simulink model "mapp_4_fir_4_str"  (R2018b)
settings: Solver=ode45  StartTime=0.0  StopTime=200  RelTol=1e-3  EnableMultiTasking=on
undefined symbols (not defined in the file or in its folder): CMD_ci_Re_0, CMD_ci_Re_21, CMD_ci_str_0, CMD_ci_str_1, CMD_ci_str_10, CMD_ci_str_11, CMD_ci_str_12, CMD_ci_str_13, CMD_ci_str_14, CMD_ci_str_15, CMD_ci_str_16, CMD_ci_str_17, CMD_ci_str_18, CMD_ci_str_19, CMD_ci_str_2, CMD_ci_str_20, CMD_ci_str_21, CMD_ci_str_3, CMD_ci_str_4, CMD_ci_str_5, CMD_ci_str_6, CMD_ci_str_7, CMD_ci_str_8, CMD_ci_str_9, CMD_decr_0, CMD_deka_down, CMD_deka_up, CMD_fb, CMD_FB_mult, CMD_Firprg_0, CMD_Firprg_1, CMD_gain, CMD_ind_mult, CMD_ind_mult_1, CMD_ind_mult_2, CMD_ind_mult_3, CMD_ind_mult_4, CMD_ind_stuk, CMD_ind_vol, CMD_ind_vol_1, CMD_ind_vol_2, CMD_ind_vol_3, CMD_ind_vol_4, CMD_init_dac, CMD_init_sw, CMD_molot_string, CMD_nl, CMD_nl_sl, CMD_omega_0, CMD_out_vol, CMD_param_0, CMD_param_5, CMD_pedal, CMD_reset, CMD_rst, CMD_shape_0, CMD_step_down, CMD_step_up, CMD_str_svertk, ind_mult_0 ... (+10)
libraries: xbsIndex_r4 x3300
(part 15 of 16)

== system mapp_4_fir_4_str/Mid_Graph2/Exp/exp-mashinka/gauss2/exp_e0 ==
  addr : Inport
  m_data : Inport  Port=2
  m_addr : Inport  Port=3
  m_en : Inport  Port=4
  Force_vol : Inport  Port=5
  AddSub5 : xbsIndex_r4/AddSub  mode=Subtraction  use_carryin=off  use_carryout=off  en=off  latency=2  precision=Full  arith_type="Signed  (2's comp)"  n_bits=24  bin_pt=0  quantization=Truncate  overflow=Wrap  use_behavioral_HDL=off  hw_selection=Fabric  pipelined=off  dbl_ovrd=off  block_type=addsub
  AddSub6 : xbsIndex_r4/AddSub  mode=Addition  use_carryin=off  use_carryout=off  en=off  latency=2  precision=Full  arith_type=Unsigned  n_bits=24  bin_pt=0  quantization=Truncate  overflow=Wrap  use_behavioral_HDL=off  hw_selection=Fabric  pipelined=off  dbl_ovrd=off  block_type=addsub
  Constant : xbsIndex_r4/Constant  const=4  gui_display_data_type=Fixed-point  arith_type=Unsigned  n_bits=3  bin_pt=0  preci_type=Single  exp_width=8  frac_width=24  explicit_period=off  period=1  equ=P=C  opselect=C  inp2=PCIN>>17  opr=+  inp1=P  carry=CIN  dbl_ovrd=off  block_type=constant
  Constant1 : xbsIndex_r4/Constant  const=0  gui_display_data_type=Fixed-point  arith_type=Unsigned  n_bits=24  bin_pt=0  preci_type=Single  exp_width=8  frac_width=24  explicit_period=on  period=1  equ=P=C  opselect=C  inp2=PCIN>>17  opr=+  inp1=P  carry=CIN  dbl_ovrd=off  block_type=constant
      settings: block_version=VER_STRING_GOES_HERE
  Constant10 : xbsIndex_r4/Constant  const=0  gui_display_data_type=Fixed-point  arith_type=Unsigned  n_bits=24  bin_pt=0  preci_type=Single  exp_width=8  frac_width=24  explicit_period=on  period=1  equ=P=C  opselect=C  inp2=PCIN>>17  opr=+  inp1=P  carry=CIN  dbl_ovrd=off  block_type=constant
      settings: block_version=VER_STRING_GOES_HERE
  Constant2 : xbsIndex_r4/Constant  const=4  gui_display_data_type=Fixed-point  arith_type=Unsigned  n_bits=3  bin_pt=0  preci_type=Single  exp_width=8  frac_width=24  explicit_period=on  period=1  equ=P=C  opselect=C  inp2=PCIN>>17  opr=+  inp1=P  carry=CIN  dbl_ovrd=off  block_type=constant
      settings: block_version=VER_STRING_GOES_HERE
  Constant3 : xbsIndex_r4/Constant  const=3  gui_display_data_type=Fixed-point  arith_type=Unsigned  n_bits=3  bin_pt=0  preci_type=Single  exp_width=8  frac_width=24  explicit_period=off  period=1  equ=P=C  opselect=C  inp2=PCIN>>17  opr=+  inp1=P  carry=CIN  dbl_ovrd=off  block_type=constant
  Constant4 : xbsIndex_r4/Constant  const=2  gui_display_data_type=Fixed-point  arith_type=Unsigned  n_bits=3  bin_pt=0  preci_type=Single  exp_width=8  frac_width=24  explicit_period=off  period=1  equ=P=C  opselect=C  inp2=PCIN>>17  opr=+  inp1=P  carry=CIN  dbl_ovrd=off  block_type=constant
  Constant5 : xbsIndex_r4/Constant  const=1  gui_display_data_type=Fixed-point  arith_type=Unsigned  n_bits=3  bin_pt=0  preci_type=Single  exp_width=8  frac_width=24  explicit_period=off  period=1  equ=P=C  opselect=C  inp2=PCIN>>17  opr=+  inp1=P  carry=CIN  dbl_ovrd=off  block_type=constant
  Constant6 : xbsIndex_r4/Constant  const=0  gui_display_data_type=Fixed-point  arith_type=Unsigned  n_bits=3  bin_pt=0  preci_type=Single  exp_width=8  frac_width=24  explicit_period=off  period=1  equ=P=C  opselect=C  inp2=PCIN>>17  opr=+  inp1=P  carry=CIN  dbl_ovrd=off  block_type=constant
  Convert5 : xbsIndex_r4/Convert  gui_display_data_type=Fixed-point  arith_type=Unsigned  n_bits=3  bin_pt=0  float_type=Single  exp_bits=8  fraction_bits=24  quantization=Truncate  overflow=Wrap  en=off  latency=0  pipeline=off  dbl_ovrd=off  block_type=convert
  Logical{,1..4} (5 alike) : xbsIndex_r4/Logical  logical_function=AND  inputs=2  en=off  latency=1  precision=Full  arith_type=Unsigned  n_bits=16  bin_pt=0  align_bp=on  dbl_ovrd=off  block_type=logical
  Mult3 : xbsIndex_r4/Mult  precision=Full  arith_type="Signed  (2's comp)"  n_bits=16  bin_pt=14  quantization=Truncate  overflow=Wrap  en=off  latency=3  use_behavioral_HDL=off  opt=Speed  use_embedded=on  optimum_pipeline=off  pipeline=on  dbl_ovrd=off  use_rpm=on  placement_style=Triangular  block_type=mult
  Mux{10..14} (5 alike) : xbsIndex_r4/Mux  inputs=2  en=off  latency=0  precision=Full  arith_type=Unsigned  n_bits=16  bin_pt=14  quantization=Truncate  overflow=Wrap  dbl_ovrd=off  block_type=mux
  Mux2 : xbsIndex_r4/Mux  inputs=2  en=off  latency=1  precision=Full  arith_type=Unsigned  n_bits=16  bin_pt=14  quantization=Truncate  overflow=Wrap  dbl_ovrd=off  block_type=mux
  Mux3 : xbsIndex_r4/Mux  inputs=5  en=off  latency=1  precision=Full  arith_type=Unsigned  n_bits=16  bin_pt=14  quantization=Truncate  overflow=Wrap  dbl_ovrd=off  block_type=mux
  Mux4 : xbsIndex_r4/Mux  inputs=5  en=off  latency=1  precision=Full  arith_type=Unsigned  n_bits=16  bin_pt=14  quantization=Truncate  overflow=Wrap  dbl_ovrd=off  block_type=mux
  RSlice1 : xbsIndex_r4/Slice  nbits=3  boolean_output=off  mode=Upper Bit Location + Width  bit1=0  base1=MSB of Input  bit0=0  base0=LSB of Input  dbl_ovrd=off  block_type=slice
      settings: block_version=VER_STRING_GOES_HERE
  RSlice7 : xbsIndex_r4/Slice  nbits=7  boolean_output=off  mode=Lower Bit Location + Width  bit1=0  base1=MSB of Input  bit0=0  base0=LSB of Input  dbl_ovrd=off  block_type=slice
      settings: block_version=VER_STRING_GOES_HERE
  Relational{1..5,16..17} (7 alike) : xbsIndex_r4/Relational  mode=a=b  op_type=Bool  en=off  latency=0  dbl_ovrd=off  block_type=relational
  Scope1 : Scope  NumInputPorts=8
  Scope2 : Scope  NumInputPorts=8
  Scope3 : Scope  NumInputPorts=10
  Shift2 : xbsIndex_r4/Shift  shift_dir=Right  shift_bits=5  en=off  latency=0  precision=Full  arith_type="Signed  (2's comp)"  n_bits=16  bin_pt=14  quantization=Truncate  overflow=Wrap  dbl_ovrd=off  block_type=shift
  Single Port RAM5 : xbsIndex_r4/Single Port RAM  depth=96  initVector=exp_e4  distributed_mem=Block RAM  write_mode=Read After Write  rst=off  init_reg=0  en=off  latency=1  optimize=Area  dbl_ovrd=off  block_type=spram
  Single Port RAM6 : xbsIndex_r4/Single Port RAM  depth=96  initVector=exp_e3  distributed_mem=Block RAM  write_mode=Read After Write  rst=off  init_reg=0  en=off  latency=1  optimize=Area  dbl_ovrd=off  block_type=spram
  Single Port RAM7 : xbsIndex_r4/Single Port RAM  depth=96  initVector=exp_e2  distributed_mem=Block RAM  write_mode=Read After Write  rst=off  init_reg=0  en=off  latency=1  optimize=Area  dbl_ovrd=off  block_type=spram
  Single Port RAM8 : xbsIndex_r4/Single Port RAM  depth=96  initVector=exp_e1  distributed_mem=Block RAM  write_mode=Read After Write  rst=off  init_reg=0  en=off  latency=1  optimize=Area  dbl_ovrd=off  block_type=spram
  Single Port RAM9 : xbsIndex_r4/Single Port RAM  depth=96  initVector=exp_e0  distributed_mem=Block RAM  write_mode=Read After Write  rst=off  init_reg=0  en=off  latency=1  optimize=Area  dbl_ovrd=off  block_type=spram
  Slice1 : xbsIndex_r4/Slice  nbits=5  boolean_output=off  mode=Lower Bit Location + Width  bit1=0  base1=LSB of Input  bit0=0  base0=LSB of Input  dbl_ovrd=off  block_type=slice
  Slice3 : xbsIndex_r4/Slice  nbits=2  boolean_output=off  mode=Upper Bit Location + Width  bit1=0  base1=MSB of Input  bit0=0  base0=LSB of Input  dbl_ovrd=off  block_type=slice
  const : xbsIndex_r4/Constant  const=0  gui_display_data_type=Fixed-point  arith_type=Unsigned  n_bits=7  bin_pt=0  preci_type=Single  exp_width=8  frac_width=24  explicit_period=on  period=1  equ=P=C  opselect=C  inp2=PCIN>>17  opr=+  inp1=P  carry=CIN  dbl_ovrd=off  block_type=constant
      settings: block_version=VER_STRING_GOES_HERE
  ind_vol_3 : xbsIndex_r4/Constant  const=CMD_ind_vol_3  gui_display_data_type=Fixed-point  arith_type=Unsigned  n_bits=8  bin_pt=0  preci_type=Single  exp_width=8  frac_width=24  explicit_period=on  period=1  equ=P=C  opselect=C  inp2=PCIN>>17  opr=+  inp1=P  carry=CIN  dbl_ovrd=off  block_type=constant
      settings: block_version=VER_STRING_GOES_HERE
  x : xbsIndex_r4/Constant  const=8000000  gui_display_data_type=Fixed-point  arith_type=Unsigned  n_bits=24  bin_pt=0  preci_type=Single  exp_width=8  frac_width=24  explicit_period=on  period=1  equ=P=C  opselect=C  inp2=PCIN>>17  opr=+  inp1=P  carry=CIN  dbl_ovrd=off  block_type=constant
      settings: block_version=VER_STRING_GOES_HERE
  z1 : xbsIndex_r4/Delay  rst=off  infoeditControl=Selection of Reset will increase slice count due to use of real FFs and instead of SRLs  en=off  latency=3  reg_retiming=on  dbl_ovrd=off  block_type=delay
      settings: block_version=8.2-EVAL
  z{2,4..13,15,17..18,20..24} (19 alike) : xbsIndex_r4/Delay  rst=off  infoeditControl=Selection of Reset will increase slice count due to use of real FFs and instead of SRLs  en=off  latency=1  reg_retiming=on  dbl_ovrd=off  block_type=delay
      settings: block_version=8.2-EVAL
  z14 : xbsIndex_r4/Delay  rst=off  infoeditControl=Selection of Reset will increase slice count due to use of real FFs and instead of SRLs  en=off  latency=2  reg_retiming=on  dbl_ovrd=off  block_type=delay
      settings: block_version=8.2-EVAL
  z3 : xbsIndex_r4/Delay  rst=off  infoeditControl=Selection of Reset will increase slice count due to use of real FFs and instead of SRLs  en=off  latency=4  reg_retiming=on  dbl_ovrd=off  block_type=delay
      settings: block_version=8.2-EVAL
  Out : Outport
  wires:
  z17/1 -> Scope1/8, Out/1
  z24/1 -> Scope1/7, AddSub6/2
  z23/1 -> Shift2/1
  z22/1 -> z21/1
  Slice1/1 -> z22/1
  z21/1 -> z20/1
  Mux2/1 -> z18/1
  z18/1 -> Scope3/1, Mux3/1, Mux4/1
  z3/1 -> z24/1
  Mux14/1 -> Single Port RAM9/1
  z4/1 -> z5/1, z6/1, z8/1, z9/1, z7/1
  Relational1/1 -> Logical/2
  Relational2/1 -> Logical1/2
  Constant1/1 -> Mux4/6
  Convert5/1 -> Mux2/2
  Mult3/1 -> z2/1
  z13/1 -> Scope3/2, Mux3/2, Mux4/3
  Relational16/1 -> Mux2/1
  Single Port RAM7/1 -> z12/1
  Single Port RAM6/1 -> z11/1
  z15/1 -> Mux4/2
  Relational5/1 -> Logical4/2
  Constant6/1 -> Relational5/2
  RSlice7/1 -> Mux10/3, Mux13/3, Mux14/3, Mux12/3, Mux11/3
  Relational17/1 -> Logical1/1, Logical2/1, Logical3/1, Logical4/1, Logical/1
  Logical1/1 -> Mux11/1, Single Port RAM6/3
  Relational3/1 -> Logical2/2
  Constant5/1 -> Relational4/2
  Slice3/1 -> Convert5/1
  Mux3/1 -> AddSub5/1, Scope3/6
  Mux12/1 -> Single Port RAM7/1
  z7/1 -> Mux12/2
  Constant4/1 -> Relational3/2
  Shift2/1 -> Scope1/3, Mult3/1
  z14/1 -> z3/1
  Mux13/1 -> Single Port RAM8/1
  m_data/1 -> Single Port RAM8/2, Single Port RAM9/2, Single Port RAM7/2, Single Port RAM6/2, Single Port RAM5/2
  Mux10/1 -> Single Port RAM5/1, Scope2/1
  z5/1 -> Mux10/2
  z6/1 -> Mux11/2
  ind_vol_3/1 -> Relational17/2
  z8/1 -> Mux13/2
  Single Port RAM5/1 -> z10/1, Scope2/3
  Constant3/1 -> Relational2/2
  Mux11/1 -> Single Port RAM6/1
  z9/1 -> Mux14/2
  Relational4/1 -> Logical3/2
  RSlice1/1 -> Relational2/1, Relational3/1, Relational4/1, Relational5/1, Relational1/1
  Logical4/1 -> Mux14/1, Single Port RAM9/3
  addr/1 -> z4/1
  Mux4/1 -> AddSub5/2, Scope3/7, z14/1
  AddSub5/1 -> z23/1
  const/1 -> Relational16/2
  z1/1 -> Scope1/4, Mult3/2
  Logical/1 -> Mux10/1, Single Port RAM5/3, Scope2/2
  Constant10/1 -> Mux3/6
  Constant/1 -> Relational1/2
  Single Port RAM9/1 -> z15/1
  z20/1 -> Scope1/2, z1/1
  Force_vol/1 -> Slice3/1, Scope1/1, Slice1/1, Relational16/1
  Logical3/1 -> Single Port RAM8/3, Mux13/1
  Single Port RAM8/1 -> z13/1
  z2/1 -> Scope1/6, AddSub6/1
  Logical2/1 -> Mux12/1, Single Port RAM7/3
  Constant2/1 -> Mux2/3
  z10/1 -> Scope3/5, Mux3/5
  m_addr/1 -> RSlice1/1, RSlice7/1
  z11/1 -> Scope3/4, Mux3/4, Mux4/5
  z12/1 -> Mux4/4, Scope3/3, Mux3/3
  m_en/1 -> Relational17/1
  AddSub6/1 -> z17/1

== system mapp_4_fir_4_str/Mid_Graph2/Exp/exp-mashinka/gauss3/exp_a0 ==
  addr : Inport
  m_data : Inport  Port=2
  m_addr : Inport  Port=3
  m_en : Inport  Port=4
  Force_vol : Inport  Port=5
  AddSub5 : xbsIndex_r4/AddSub  mode=Subtraction  use_carryin=off  use_carryout=off  en=off  latency=2  precision=Full  arith_type="Signed  (2's comp)"  n_bits=24  bin_pt=0  quantization=Truncate  overflow=Wrap  use_behavioral_HDL=off  hw_selection=Fabric  pipelined=off  dbl_ovrd=off  block_type=addsub
  AddSub6 : xbsIndex_r4/AddSub  mode=Addition  use_carryin=off  use_carryout=off  en=off  latency=2  precision=Full  arith_type=Unsigned  n_bits=24  bin_pt=0  quantization=Truncate  overflow=Wrap  use_behavioral_HDL=off  hw_selection=Fabric  pipelined=off  dbl_ovrd=off  block_type=addsub
  CMD_step_down : xbsIndex_r4/Constant  const=CMD_step_down  gui_display_data_type=Fixed-point  arith_type=Unsigned  n_bits=8  bin_pt=0  preci_type=Single  exp_width=8  frac_width=24  explicit_period=on  period=1  equ=P=C  opselect=C  inp2=PCIN>>17  opr=+  inp1=P  carry=CIN  dbl_ovrd=off  block_type=constant
      settings: block_version=VER_STRING_GOES_HERE
  Constant : xbsIndex_r4/Constant  const=4  gui_display_data_type=Fixed-point  arith_type=Unsigned  n_bits=3  bin_pt=0  preci_type=Single  exp_width=8  frac_width=24  explicit_period=off  period=1  equ=P=C  opselect=C  inp2=PCIN>>17  opr=+  inp1=P  carry=CIN  dbl_ovrd=off  block_type=constant
  Constant1 : xbsIndex_r4/Constant  const=0  gui_display_data_type=Fixed-point  arith_type=Unsigned  n_bits=24  bin_pt=0  preci_type=Single  exp_width=8  frac_width=24  explicit_period=on  period=1  equ=P=C  opselect=C  inp2=PCIN>>17  opr=+  inp1=P  carry=CIN  dbl_ovrd=off  block_type=constant
      settings: block_version=VER_STRING_GOES_HERE
  Constant10 : xbsIndex_r4/Constant  const=0  gui_display_data_type=Fixed-point  arith_type=Unsigned  n_bits=24  bin_pt=0  preci_type=Single  exp_width=8  frac_width=24  explicit_period=on  period=1  equ=P=C  opselect=C  inp2=PCIN>>17  opr=+  inp1=P  carry=CIN  dbl_ovrd=off  block_type=constant
      settings: block_version=VER_STRING_GOES_HERE
  Constant2 : xbsIndex_r4/Constant  const=4  gui_display_data_type=Fixed-point  arith_type=Unsigned  n_bits=3  bin_pt=0  preci_type=Single  exp_width=8  frac_width=24  explicit_period=on  period=1  equ=P=C  opselect=C  inp2=PCIN>>17  opr=+  inp1=P  carry=CIN  dbl_ovrd=off  block_type=constant
      settings: block_version=VER_STRING_GOES_HERE
  Constant3 : xbsIndex_r4/Constant  const=3  gui_display_data_type=Fixed-point  arith_type=Unsigned  n_bits=3  bin_pt=0  preci_type=Single  exp_width=8  frac_width=24  explicit_period=off  period=1  equ=P=C  opselect=C  inp2=PCIN>>17  opr=+  inp1=P  carry=CIN  dbl_ovrd=off  block_type=constant
  Constant4 : xbsIndex_r4/Constant  const=2  gui_display_data_type=Fixed-point  arith_type=Unsigned  n_bits=3  bin_pt=0  preci_type=Single  exp_width=8  frac_width=24  explicit_period=off  period=1  equ=P=C  opselect=C  inp2=PCIN>>17  opr=+  inp1=P  carry=CIN  dbl_ovrd=off  block_type=constant
  Constant5 : xbsIndex_r4/Constant  const=1  gui_display_data_type=Fixed-point  arith_type=Unsigned  n_bits=3  bin_pt=0  preci_type=Single  exp_width=8  frac_width=24  explicit_period=off  period=1  equ=P=C  opselect=C  inp2=PCIN>>17  opr=+  inp1=P  carry=CIN  dbl_ovrd=off  block_type=constant
  Constant6 : xbsIndex_r4/Constant  const=0  gui_display_data_type=Fixed-point  arith_type=Unsigned  n_bits=3  bin_pt=0  preci_type=Single  exp_width=8  frac_width=24  explicit_period=off  period=1  equ=P=C  opselect=C  inp2=PCIN>>17  opr=+  inp1=P  carry=CIN  dbl_ovrd=off  block_type=constant
  Convert5 : xbsIndex_r4/Convert  gui_display_data_type=Fixed-point  arith_type=Unsigned  n_bits=3  bin_pt=0  float_type=Single  exp_bits=8  fraction_bits=24  quantization=Truncate  overflow=Wrap  en=off  latency=0  pipeline=off  dbl_ovrd=off  block_type=convert
  Logical{,1..4} (5 alike) : xbsIndex_r4/Logical  logical_function=AND  inputs=2  en=off  latency=1  precision=Full  arith_type=Unsigned  n_bits=16  bin_pt=0  align_bp=on  dbl_ovrd=off  block_type=logical
  Mult3 : xbsIndex_r4/Mult  precision=Full  arith_type="Signed  (2's comp)"  n_bits=16  bin_pt=14  quantization=Truncate  overflow=Wrap  en=off  latency=3  use_behavioral_HDL=off  opt=Speed  use_embedded=on  optimum_pipeline=off  pipeline=on  dbl_ovrd=off  use_rpm=on  placement_style=Triangular  block_type=mult
  Mux{10..14} (5 alike) : xbsIndex_r4/Mux  inputs=2  en=off  latency=0  precision=Full  arith_type=Unsigned  n_bits=16  bin_pt=14  quantization=Truncate  overflow=Wrap  dbl_ovrd=off  block_type=mux
  Mux2 : xbsIndex_r4/Mux  inputs=2  en=off  latency=1  precision=Full  arith_type=Unsigned  n_bits=16  bin_pt=14  quantization=Truncate  overflow=Wrap  dbl_ovrd=off  block_type=mux
  Mux3 : xbsIndex_r4/Mux  inputs=5  en=off  latency=1  precision=Full  arith_type=Unsigned  n_bits=16  bin_pt=14  quantization=Truncate  overflow=Wrap  dbl_ovrd=off  block_type=mux
  Mux4 : xbsIndex_r4/Mux  inputs=5  en=off  latency=1  precision=Full  arith_type=Unsigned  n_bits=16  bin_pt=14  quantization=Truncate  overflow=Wrap  dbl_ovrd=off  block_type=mux
  RSlice1 : xbsIndex_r4/Slice  nbits=3  boolean_output=off  mode=Upper Bit Location + Width  bit1=0  base1=MSB of Input  bit0=0  base0=LSB of Input  dbl_ovrd=off  block_type=slice
      settings: block_version=VER_STRING_GOES_HERE
  RSlice7 : xbsIndex_r4/Slice  nbits=7  boolean_output=off  mode=Lower Bit Location + Width  bit1=0  base1=MSB of Input  bit0=0  base0=LSB of Input  dbl_ovrd=off  block_type=slice
      settings: block_version=VER_STRING_GOES_HERE
  Relational{1..5,16..17} (7 alike) : xbsIndex_r4/Relational  mode=a=b  op_type=Bool  en=off  latency=0  dbl_ovrd=off  block_type=relational
  Scope1 : Scope  NumInputPorts=8
  Scope2 : Scope  NumInputPorts=8
  Scope3 : Scope  NumInputPorts=10
  Shift2 : xbsIndex_r4/Shift  shift_dir=Right  shift_bits=5  en=off  latency=0  precision=Full  arith_type="Signed  (2's comp)"  n_bits=16  bin_pt=14  quantization=Truncate  overflow=Wrap  dbl_ovrd=off  block_type=shift
  Single Port RAM5 : xbsIndex_r4/Single Port RAM  depth=96  initVector=exp_a4  distributed_mem=Block RAM  write_mode=Read After Write  rst=off  init_reg=0  en=off  latency=1  optimize=Area  dbl_ovrd=off  block_type=spram
  Single Port RAM6 : xbsIndex_r4/Single Port RAM  depth=96  initVector=exp_a3  distributed_mem=Block RAM  write_mode=Read After Write  rst=off  init_reg=0  en=off  latency=1  optimize=Area  dbl_ovrd=off  block_type=spram
  Single Port RAM7 : xbsIndex_r4/Single Port RAM  depth=96  initVector=exp_a2  distributed_mem=Block RAM  write_mode=Read After Write  rst=off  init_reg=0  en=off  latency=1  optimize=Area  dbl_ovrd=off  block_type=spram
  Single Port RAM8 : xbsIndex_r4/Single Port RAM  depth=96  initVector=exp_a1  distributed_mem=Block RAM  write_mode=Read After Write  rst=off  init_reg=0  en=off  latency=1  optimize=Area  dbl_ovrd=off  block_type=spram
  Single Port RAM9 : xbsIndex_r4/Single Port RAM  depth=96  initVector=exp_a0  distributed_mem=Block RAM  write_mode=Read After Write  rst=off  init_reg=0  en=off  latency=1  optimize=Area  dbl_ovrd=off  block_type=spram
  Slice1 : xbsIndex_r4/Slice  nbits=5  boolean_output=off  mode=Lower Bit Location + Width  bit1=0  base1=LSB of Input  bit0=0  base0=LSB of Input  dbl_ovrd=off  block_type=slice
  Slice3 : xbsIndex_r4/Slice  nbits=2  boolean_output=off  mode=Upper Bit Location + Width  bit1=0  base1=MSB of Input  bit0=0  base0=LSB of Input  dbl_ovrd=off  block_type=slice
  const : xbsIndex_r4/Constant  const=0  gui_display_data_type=Fixed-point  arith_type=Unsigned  n_bits=7  bin_pt=0  preci_type=Single  exp_width=8  frac_width=24  explicit_period=on  period=1  equ=P=C  opselect=C  inp2=PCIN>>17  opr=+  inp1=P  carry=CIN  dbl_ovrd=off  block_type=constant
      settings: block_version=VER_STRING_GOES_HERE
  x : xbsIndex_r4/Constant  const=8000000  gui_display_data_type=Fixed-point  arith_type=Unsigned  n_bits=24  bin_pt=0  preci_type=Single  exp_width=8  frac_width=24  explicit_period=on  period=1  equ=P=C  opselect=C  inp2=PCIN>>17  opr=+  inp1=P  carry=CIN  dbl_ovrd=off  block_type=constant
      settings: block_version=VER_STRING_GOES_HERE
  z1 : xbsIndex_r4/Delay  rst=off  infoeditControl=Selection of Reset will increase slice count due to use of real FFs and instead of SRLs  en=off  latency=3  reg_retiming=on  dbl_ovrd=off  block_type=delay
      settings: block_version=8.2-EVAL
  z{2,4..13,15,17..18,20..24} (19 alike) : xbsIndex_r4/Delay  rst=off  infoeditControl=Selection of Reset will increase slice count due to use of real FFs and instead of SRLs  en=off  latency=1  reg_retiming=on  dbl_ovrd=off  block_type=delay
      settings: block_version=8.2-EVAL
  z14 : xbsIndex_r4/Delay  rst=off  infoeditControl=Selection of Reset will increase slice count due to use of real FFs and instead of SRLs  en=off  latency=2  reg_retiming=on  dbl_ovrd=off  block_type=delay
      settings: block_version=8.2-EVAL
  z3 : xbsIndex_r4/Delay  rst=off  infoeditControl=Selection of Reset will increase slice count due to use of real FFs and instead of SRLs  en=off  latency=4  reg_retiming=on  dbl_ovrd=off  block_type=delay
      settings: block_version=8.2-EVAL
  Out : Outport
  wires:
  AddSub6/1 -> z17/1
  m_en/1 -> Relational17/1
  z12/1 -> Mux3/3, Scope3/3, Mux4/4
  z11/1 -> Mux4/5, Mux3/4, Scope3/4
  m_addr/1 -> RSlice7/1, RSlice1/1
  z10/1 -> Mux3/5, Scope3/5
  Constant2/1 -> Mux2/3
  Logical2/1 -> Single Port RAM7/3, Mux12/1
  z2/1 -> Scope1/4, AddSub6/1
  Single Port RAM8/1 -> z13/1
  Logical3/1 -> Mux13/1, Single Port RAM8/3
  Force_vol/1 -> Relational16/1, Slice1/1, Slice3/1
  z20/1 -> z1/1
  Single Port RAM9/1 -> z15/1
  Constant/1 -> Relational1/2
  Constant10/1 -> Mux3/6
  Logical/1 -> Scope2/2, Single Port RAM5/3, Mux10/1
  z1/1 -> Scope1/3, Mult3/2
  const/1 -> Relational16/2
  AddSub5/1 -> z23/1
  Mux4/1 -> z14/1, Scope3/7, AddSub5/2
  addr/1 -> z4/1
  Logical4/1 -> Single Port RAM9/3, Mux14/1
  RSlice1/1 -> Relational1/1, Relational5/1, Relational4/1, Relational3/1, Relational2/1
  Relational4/1 -> Logical3/2
  z9/1 -> Mux14/2
  Mux11/1 -> Single Port RAM6/1
  Constant3/1 -> Relational2/2
  Single Port RAM5/1 -> Scope2/3, z10/1
  z8/1 -> Mux13/2
  CMD_step_down/1 -> Relational17/2
  z6/1 -> Mux11/2
  z5/1 -> Mux10/2
  Mux10/1 -> Scope2/1, Single Port RAM5/1
  m_data/1 -> Single Port RAM5/2, Single Port RAM6/2, Single Port RAM7/2, Single Port RAM9/2, Single Port RAM8/2
  Mux13/1 -> Single Port RAM8/1
  z14/1 -> z3/1
  Shift2/1 -> Scope1/1, Mult3/1
  Constant4/1 -> Relational3/2
  z7/1 -> Mux12/2
  Mux12/1 -> Single Port RAM7/1
  Mux3/1 -> Scope3/6, AddSub5/1
  Slice3/1 -> Convert5/1
  Constant5/1 -> Relational4/2
  Relational3/1 -> Logical2/2
  Logical1/1 -> Single Port RAM6/3, Mux11/1
  Relational17/1 -> Logical/1, Logical4/1, Logical3/1, Logical2/1, Logical1/1
  RSlice7/1 -> Mux11/3, Mux12/3, Mux14/3, Mux13/3, Mux10/3
  Constant6/1 -> Relational5/2
  Relational5/1 -> Logical4/2
  z15/1 -> Mux4/2
  Single Port RAM6/1 -> z11/1
  Single Port RAM7/1 -> z12/1
  Relational16/1 -> Mux2/1
  z13/1 -> Mux4/3, Mux3/2, Scope3/2
  Mult3/1 -> z2/1
  Convert5/1 -> Mux2/2
  Constant1/1 -> Mux4/6
  Relational2/1 -> Logical1/2
  Relational1/1 -> Logical/2
  z4/1 -> z7/1, z9/1, z8/1, z6/1, z5/1
  Mux14/1 -> Single Port RAM9/1
  z3/1 -> z24/1
  z18/1 -> Mux4/1, Mux3/1, Scope3/1
  Mux2/1 -> z18/1
  z21/1 -> z20/1
  Slice1/1 -> z22/1
  z22/1 -> z21/1
  z23/1 -> Shift2/1
  z24/1 -> Scope1/5, AddSub6/2
  z17/1 -> Scope1/6, Out/1

== system mapp_4_fir_4_str/Mid_Graph2/Exp/exp-mashinka/gauss3/exp_d0 ==
  addr : Inport
  m_data : Inport  Port=2
  m_addr : Inport  Port=3
  m_en : Inport  Port=4
  Force_vol : Inport  Port=5
  AddSub5 : xbsIndex_r4/AddSub  mode=Subtraction  use_carryin=off  use_carryout=off  en=off  latency=2  precision=Full  arith_type="Signed  (2's comp)"  n_bits=24  bin_pt=0  quantization=Truncate  overflow=Wrap  use_behavioral_HDL=off  hw_selection=Fabric  pipelined=off  dbl_ovrd=off  block_type=addsub
  AddSub6 : xbsIndex_r4/AddSub  mode=Addition  use_carryin=off  use_carryout=off  en=off  latency=2  precision=Full  arith_type=Unsigned  n_bits=24  bin_pt=0  quantization=Truncate  overflow=Wrap  use_behavioral_HDL=off  hw_selection=Fabric  pipelined=off  dbl_ovrd=off  block_type=addsub
  CMD_step_up : xbsIndex_r4/Constant  const=CMD_step_up  gui_display_data_type=Fixed-point  arith_type=Unsigned  n_bits=8  bin_pt=0  preci_type=Single  exp_width=8  frac_width=24  explicit_period=on  period=1  equ=P=C  opselect=C  inp2=PCIN>>17  opr=+  inp1=P  carry=CIN  dbl_ovrd=off  block_type=constant
      settings: block_version=VER_STRING_GOES_HERE
  Constant : xbsIndex_r4/Constant  const=4  gui_display_data_type=Fixed-point  arith_type=Unsigned  n_bits=3  bin_pt=0  preci_type=Single  exp_width=8  frac_width=24  explicit_period=off  period=1  equ=P=C  opselect=C  inp2=PCIN>>17  opr=+  inp1=P  carry=CIN  dbl_ovrd=off  block_type=constant
  Constant1 : xbsIndex_r4/Constant  const=0  gui_display_data_type=Fixed-point  arith_type=Unsigned  n_bits=24  bin_pt=0  preci_type=Single  exp_width=8  frac_width=24  explicit_period=on  period=1  equ=P=C  opselect=C  inp2=PCIN>>17  opr=+  inp1=P  carry=CIN  dbl_ovrd=off  block_type=constant
      settings: block_version=VER_STRING_GOES_HERE
  Constant10 : xbsIndex_r4/Constant  const=0  gui_display_data_type=Fixed-point  arith_type=Unsigned  n_bits=24  bin_pt=0  preci_type=Single  exp_width=8  frac_width=24  explicit_period=on  period=1  equ=P=C  opselect=C  inp2=PCIN>>17  opr=+  inp1=P  carry=CIN  dbl_ovrd=off  block_type=constant
      settings: block_version=VER_STRING_GOES_HERE
  Constant2 : xbsIndex_r4/Constant  const=4  gui_display_data_type=Fixed-point  arith_type=Unsigned  n_bits=3  bin_pt=0  preci_type=Single  exp_width=8  frac_width=24  explicit_period=on  period=1  equ=P=C  opselect=C  inp2=PCIN>>17  opr=+  inp1=P  carry=CIN  dbl_ovrd=off  block_type=constant
      settings: block_version=VER_STRING_GOES_HERE
  Constant3 : xbsIndex_r4/Constant  const=3  gui_display_data_type=Fixed-point  arith_type=Unsigned  n_bits=3  bin_pt=0  preci_type=Single  exp_width=8  frac_width=24  explicit_period=off  period=1  equ=P=C  opselect=C  inp2=PCIN>>17  opr=+  inp1=P  carry=CIN  dbl_ovrd=off  block_type=constant
  Constant4 : xbsIndex_r4/Constant  const=2  gui_display_data_type=Fixed-point  arith_type=Unsigned  n_bits=3  bin_pt=0  preci_type=Single  exp_width=8  frac_width=24  explicit_period=off  period=1  equ=P=C  opselect=C  inp2=PCIN>>17  opr=+  inp1=P  carry=CIN  dbl_ovrd=off  block_type=constant
  Constant5 : xbsIndex_r4/Constant  const=1  gui_display_data_type=Fixed-point  arith_type=Unsigned  n_bits=3  bin_pt=0  preci_type=Single  exp_width=8  frac_width=24  explicit_period=off  period=1  equ=P=C  opselect=C  inp2=PCIN>>17  opr=+  inp1=P  carry=CIN  dbl_ovrd=off  block_type=constant
  Constant6 : xbsIndex_r4/Constant  const=0  gui_display_data_type=Fixed-point  arith_type=Unsigned  n_bits=3  bin_pt=0  preci_type=Single  exp_width=8  frac_width=24  explicit_period=off  period=1  equ=P=C  opselect=C  inp2=PCIN>>17  opr=+  inp1=P  carry=CIN  dbl_ovrd=off  block_type=constant
  Convert5 : xbsIndex_r4/Convert  gui_display_data_type=Fixed-point  arith_type=Unsigned  n_bits=3  bin_pt=0  float_type=Single  exp_bits=8  fraction_bits=24  quantization=Truncate  overflow=Wrap  en=off  latency=0  pipeline=off  dbl_ovrd=off  block_type=convert
  Logical{,1..4} (5 alike) : xbsIndex_r4/Logical  logical_function=AND  inputs=2  en=off  latency=1  precision=Full  arith_type=Unsigned  n_bits=16  bin_pt=0  align_bp=on  dbl_ovrd=off  block_type=logical
  Mult3 : xbsIndex_r4/Mult  precision=Full  arith_type="Signed  (2's comp)"  n_bits=16  bin_pt=14  quantization=Truncate  overflow=Wrap  en=off  latency=3  use_behavioral_HDL=off  opt=Speed  use_embedded=on  optimum_pipeline=off  pipeline=on  dbl_ovrd=off  use_rpm=on  placement_style=Triangular  block_type=mult
  Mux{10..14} (5 alike) : xbsIndex_r4/Mux  inputs=2  en=off  latency=0  precision=Full  arith_type=Unsigned  n_bits=16  bin_pt=14  quantization=Truncate  overflow=Wrap  dbl_ovrd=off  block_type=mux
  Mux2 : xbsIndex_r4/Mux  inputs=2  en=off  latency=1  precision=Full  arith_type=Unsigned  n_bits=16  bin_pt=14  quantization=Truncate  overflow=Wrap  dbl_ovrd=off  block_type=mux
  Mux3 : xbsIndex_r4/Mux  inputs=5  en=off  latency=1  precision=Full  arith_type=Unsigned  n_bits=16  bin_pt=14  quantization=Truncate  overflow=Wrap  dbl_ovrd=off  block_type=mux
  Mux4 : xbsIndex_r4/Mux  inputs=5  en=off  latency=1  precision=Full  arith_type=Unsigned  n_bits=16  bin_pt=14  quantization=Truncate  overflow=Wrap  dbl_ovrd=off  block_type=mux
  RSlice1 : xbsIndex_r4/Slice  nbits=3  boolean_output=off  mode=Upper Bit Location + Width  bit1=0  base1=MSB of Input  bit0=0  base0=LSB of Input  dbl_ovrd=off  block_type=slice
      settings: block_version=VER_STRING_GOES_HERE
  RSlice7 : xbsIndex_r4/Slice  nbits=7  boolean_output=off  mode=Lower Bit Location + Width  bit1=0  base1=MSB of Input  bit0=0  base0=LSB of Input  dbl_ovrd=off  block_type=slice
      settings: block_version=VER_STRING_GOES_HERE
  Relational{1..5,16..17} (7 alike) : xbsIndex_r4/Relational  mode=a=b  op_type=Bool  en=off  latency=0  dbl_ovrd=off  block_type=relational
  Scope1 : Scope  NumInputPorts=8
  Scope2 : Scope  NumInputPorts=8
  Scope3 : Scope  NumInputPorts=10
  Shift2 : xbsIndex_r4/Shift  shift_dir=Right  shift_bits=5  en=off  latency=0  precision=Full  arith_type="Signed  (2's comp)"  n_bits=16  bin_pt=14  quantization=Truncate  overflow=Wrap  dbl_ovrd=off  block_type=shift
  Single Port RAM5 : xbsIndex_r4/Single Port RAM  depth=96  initVector=exp_d4  distributed_mem=Block RAM  write_mode=Read After Write  rst=off  init_reg=0  en=off  latency=1  optimize=Area  dbl_ovrd=off  block_type=spram
  Single Port RAM6 : xbsIndex_r4/Single Port RAM  depth=96  initVector=exp_d3  distributed_mem=Block RAM  write_mode=Read After Write  rst=off  init_reg=0  en=off  latency=1  optimize=Area  dbl_ovrd=off  block_type=spram
  Single Port RAM7 : xbsIndex_r4/Single Port RAM  depth=96  initVector=exp_d2  distributed_mem=Block RAM  write_mode=Read After Write  rst=off  init_reg=0  en=off  latency=1  optimize=Area  dbl_ovrd=off  block_type=spram
  Single Port RAM8 : xbsIndex_r4/Single Port RAM  depth=96  initVector=exp_d1  distributed_mem=Block RAM  write_mode=Read After Write  rst=off  init_reg=0  en=off  latency=1  optimize=Area  dbl_ovrd=off  block_type=spram
  Single Port RAM9 : xbsIndex_r4/Single Port RAM  depth=96  initVector=exp_d0  distributed_mem=Block RAM  write_mode=Read After Write  rst=off  init_reg=0  en=off  latency=1  optimize=Area  dbl_ovrd=off  block_type=spram
  Slice1 : xbsIndex_r4/Slice  nbits=5  boolean_output=off  mode=Lower Bit Location + Width  bit1=0  base1=LSB of Input  bit0=0  base0=LSB of Input  dbl_ovrd=off  block_type=slice
  Slice3 : xbsIndex_r4/Slice  nbits=2  boolean_output=off  mode=Upper Bit Location + Width  bit1=0  base1=MSB of Input  bit0=0  base0=LSB of Input  dbl_ovrd=off  block_type=slice
  const : xbsIndex_r4/Constant  const=0  gui_display_data_type=Fixed-point  arith_type=Unsigned  n_bits=7  bin_pt=0  preci_type=Single  exp_width=8  frac_width=24  explicit_period=on  period=1  equ=P=C  opselect=C  inp2=PCIN>>17  opr=+  inp1=P  carry=CIN  dbl_ovrd=off  block_type=constant
      settings: block_version=VER_STRING_GOES_HERE
  x : xbsIndex_r4/Constant  const=8000000  gui_display_data_type=Fixed-point  arith_type=Unsigned  n_bits=24  bin_pt=0  preci_type=Single  exp_width=8  frac_width=24  explicit_period=on  period=1  equ=P=C  opselect=C  inp2=PCIN>>17  opr=+  inp1=P  carry=CIN  dbl_ovrd=off  block_type=constant
      settings: block_version=VER_STRING_GOES_HERE
  z1 : xbsIndex_r4/Delay  rst=off  infoeditControl=Selection of Reset will increase slice count due to use of real FFs and instead of SRLs  en=off  latency=3  reg_retiming=on  dbl_ovrd=off  block_type=delay
      settings: block_version=8.2-EVAL
  z{2,4..13,15,17..18,20..24} (19 alike) : xbsIndex_r4/Delay  rst=off  infoeditControl=Selection of Reset will increase slice count due to use of real FFs and instead of SRLs  en=off  latency=1  reg_retiming=on  dbl_ovrd=off  block_type=delay
      settings: block_version=8.2-EVAL
  z14 : xbsIndex_r4/Delay  rst=off  infoeditControl=Selection of Reset will increase slice count due to use of real FFs and instead of SRLs  en=off  latency=2  reg_retiming=on  dbl_ovrd=off  block_type=delay
      settings: block_version=8.2-EVAL
  z3 : xbsIndex_r4/Delay  rst=off  infoeditControl=Selection of Reset will increase slice count due to use of real FFs and instead of SRLs  en=off  latency=4  reg_retiming=on  dbl_ovrd=off  block_type=delay
      settings: block_version=8.2-EVAL
  Out : Outport
  wires:
  z17/1 -> Out/1, Scope1/6
  z24/1 -> AddSub6/2, Scope1/5
  z23/1 -> Shift2/1
  z22/1 -> z21/1
  Slice1/1 -> z22/1
  z21/1 -> z20/1
  Mux2/1 -> z18/1
  z18/1 -> Scope3/1, Mux3/1, Mux4/1
  z3/1 -> z24/1
  Mux14/1 -> Single Port RAM9/1
  z4/1 -> z5/1, z6/1, z8/1, z9/1, z7/1
  Relational1/1 -> Logical/2
  Relational2/1 -> Logical1/2
  Constant1/1 -> Mux4/6
  Convert5/1 -> Mux2/2
  Mult3/1 -> z2/1
  z13/1 -> Scope3/2, Mux3/2, Mux4/3
  Relational16/1 -> Mux2/1
  Single Port RAM7/1 -> z12/1
  Single Port RAM6/1 -> z11/1
  z15/1 -> Mux4/2
  Relational5/1 -> Logical4/2
  Constant6/1 -> Relational5/2
  RSlice7/1 -> Mux10/3, Mux13/3, Mux14/3, Mux12/3, Mux11/3
  Relational17/1 -> Logical1/1, Logical2/1, Logical3/1, Logical4/1, Logical/1
  Logical1/1 -> Mux11/1, Single Port RAM6/3
  Relational3/1 -> Logical2/2
  Constant5/1 -> Relational4/2
  Slice3/1 -> Convert5/1
  Mux3/1 -> AddSub5/1, Scope3/6
  Mux12/1 -> Single Port RAM7/1
  z7/1 -> Mux12/2
  Constant4/1 -> Relational3/2
  Shift2/1 -> Mult3/1, Scope1/1
  z14/1 -> z3/1
  Mux13/1 -> Single Port RAM8/1
  m_data/1 -> Single Port RAM8/2, Single Port RAM9/2, Single Port RAM7/2, Single Port RAM6/2, Single Port RAM5/2
  Mux10/1 -> Single Port RAM5/1, Scope2/1
  z5/1 -> Mux10/2
  z6/1 -> Mux11/2
  CMD_step_up/1 -> Relational17/2
  z8/1 -> Mux13/2
  Single Port RAM5/1 -> z10/1, Scope2/3
  Constant3/1 -> Relational2/2
  Mux11/1 -> Single Port RAM6/1
  z9/1 -> Mux14/2
  Relational4/1 -> Logical3/2
  RSlice1/1 -> Relational2/1, Relational3/1, Relational4/1, Relational5/1, Relational1/1
  Logical4/1 -> Mux14/1, Single Port RAM9/3
  addr/1 -> z4/1
  Mux4/1 -> AddSub5/2, Scope3/7, z14/1
  AddSub5/1 -> z23/1
  const/1 -> Relational16/2
  z1/1 -> Mult3/2, Scope1/3
  Logical/1 -> Mux10/1, Single Port RAM5/3, Scope2/2
  Constant10/1 -> Mux3/6
  Constant/1 -> Relational1/2
  Single Port RAM9/1 -> z15/1
  z20/1 -> z1/1, Scope1/2
  Force_vol/1 -> Slice3/1, Slice1/1, Relational16/1
  Logical3/1 -> Single Port RAM8/3, Mux13/1
  Single Port RAM8/1 -> z13/1
  z2/1 -> AddSub6/1, Scope1/4
  Logical2/1 -> Mux12/1, Single Port RAM7/3
  Constant2/1 -> Mux2/3
  z10/1 -> Scope3/5, Mux3/5
  m_addr/1 -> RSlice1/1, RSlice7/1
  z11/1 -> Scope3/4, Mux3/4, Mux4/5
  z12/1 -> Mux4/4, Scope3/3, Mux3/3
  m_en/1 -> Relational17/1
  AddSub6/1 -> z17/1

== system mapp_4_fir_4_str/Mid_Graph2/Exp/exp-mashinka/gauss3/exp_e0 ==
  addr : Inport
  m_data : Inport  Port=2
  m_addr : Inport  Port=3
  m_en : Inport  Port=4
  Force_vol : Inport  Port=5
  AddSub5 : xbsIndex_r4/AddSub  mode=Subtraction  use_carryin=off  use_carryout=off  en=off  latency=2  precision=Full  arith_type="Signed  (2's comp)"  n_bits=24  bin_pt=0  quantization=Truncate  overflow=Wrap  use_behavioral_HDL=off  hw_selection=Fabric  pipelined=off  dbl_ovrd=off  block_type=addsub
  AddSub6 : xbsIndex_r4/AddSub  mode=Addition  use_carryin=off  use_carryout=off  en=off  latency=2  precision=Full  arith_type=Unsigned  n_bits=24  bin_pt=0  quantization=Truncate  overflow=Wrap  use_behavioral_HDL=off  hw_selection=Fabric  pipelined=off  dbl_ovrd=off  block_type=addsub
  CMD_Firprg_1 : xbsIndex_r4/Constant  const=CMD_Firprg_1  gui_display_data_type=Fixed-point  arith_type=Unsigned  n_bits=8  bin_pt=0  preci_type=Single  exp_width=8  frac_width=24  explicit_period=on  period=1  equ=P=C  opselect=C  inp2=PCIN>>17  opr=+  inp1=P  carry=CIN  dbl_ovrd=off  block_type=constant
      settings: block_version=VER_STRING_GOES_HERE
  Constant : xbsIndex_r4/Constant  const=4  gui_display_data_type=Fixed-point  arith_type=Unsigned  n_bits=3  bin_pt=0  preci_type=Single  exp_width=8  frac_width=24  explicit_period=off  period=1  equ=P=C  opselect=C  inp2=PCIN>>17  opr=+  inp1=P  carry=CIN  dbl_ovrd=off  block_type=constant
  Constant1 : xbsIndex_r4/Constant  const=0  gui_display_data_type=Fixed-point  arith_type=Unsigned  n_bits=24  bin_pt=0  preci_type=Single  exp_width=8  frac_width=24  explicit_period=on  period=1  equ=P=C  opselect=C  inp2=PCIN>>17  opr=+  inp1=P  carry=CIN  dbl_ovrd=off  block_type=constant
      settings: block_version=VER_STRING_GOES_HERE
  Constant10 : xbsIndex_r4/Constant  const=0  gui_display_data_type=Fixed-point  arith_type=Unsigned  n_bits=24  bin_pt=0  preci_type=Single  exp_width=8  frac_width=24  explicit_period=on  period=1  equ=P=C  opselect=C  inp2=PCIN>>17  opr=+  inp1=P  carry=CIN  dbl_ovrd=off  block_type=constant
      settings: block_version=VER_STRING_GOES_HERE
  Constant2 : xbsIndex_r4/Constant  const=4  gui_display_data_type=Fixed-point  arith_type=Unsigned  n_bits=3  bin_pt=0  preci_type=Single  exp_width=8  frac_width=24  explicit_period=on  period=1  equ=P=C  opselect=C  inp2=PCIN>>17  opr=+  inp1=P  carry=CIN  dbl_ovrd=off  block_type=constant
      settings: block_version=VER_STRING_GOES_HERE
  Constant3 : xbsIndex_r4/Constant  const=3  gui_display_data_type=Fixed-point  arith_type=Unsigned  n_bits=3  bin_pt=0  preci_type=Single  exp_width=8  frac_width=24  explicit_period=off  period=1  equ=P=C  opselect=C  inp2=PCIN>>17  opr=+  inp1=P  carry=CIN  dbl_ovrd=off  block_type=constant
  Constant4 : xbsIndex_r4/Constant  const=2  gui_display_data_type=Fixed-point  arith_type=Unsigned  n_bits=3  bin_pt=0  preci_type=Single  exp_width=8  frac_width=24  explicit_period=off  period=1  equ=P=C  opselect=C  inp2=PCIN>>17  opr=+  inp1=P  carry=CIN  dbl_ovrd=off  block_type=constant
  Constant5 : xbsIndex_r4/Constant  const=1  gui_display_data_type=Fixed-point  arith_type=Unsigned  n_bits=3  bin_pt=0  preci_type=Single  exp_width=8  frac_width=24  explicit_period=off  period=1  equ=P=C  opselect=C  inp2=PCIN>>17  opr=+  inp1=P  carry=CIN  dbl_ovrd=off  block_type=constant
  Constant6 : xbsIndex_r4/Constant  const=0  gui_display_data_type=Fixed-point  arith_type=Unsigned  n_bits=3  bin_pt=0  preci_type=Single  exp_width=8  frac_width=24  explicit_period=off  period=1  equ=P=C  opselect=C  inp2=PCIN>>17  opr=+  inp1=P  carry=CIN  dbl_ovrd=off  block_type=constant
  Convert5 : xbsIndex_r4/Convert  gui_display_data_type=Fixed-point  arith_type=Unsigned  n_bits=3  bin_pt=0  float_type=Single  exp_bits=8  fraction_bits=24  quantization=Truncate  overflow=Wrap  en=off  latency=0  pipeline=off  dbl_ovrd=off  block_type=convert
  Logical{,1..4} (5 alike) : xbsIndex_r4/Logical  logical_function=AND  inputs=2  en=off  latency=1  precision=Full  arith_type=Unsigned  n_bits=16  bin_pt=0  align_bp=on  dbl_ovrd=off  block_type=logical
  Mult3 : xbsIndex_r4/Mult  precision=Full  arith_type="Signed  (2's comp)"  n_bits=16  bin_pt=14  quantization=Truncate  overflow=Wrap  en=off  latency=3  use_behavioral_HDL=off  opt=Speed  use_embedded=on  optimum_pipeline=off  pipeline=on  dbl_ovrd=off  use_rpm=on  placement_style=Triangular  block_type=mult
  Mux{10..14} (5 alike) : xbsIndex_r4/Mux  inputs=2  en=off  latency=0  precision=Full  arith_type=Unsigned  n_bits=16  bin_pt=14  quantization=Truncate  overflow=Wrap  dbl_ovrd=off  block_type=mux
  Mux2 : xbsIndex_r4/Mux  inputs=2  en=off  latency=1  precision=Full  arith_type=Unsigned  n_bits=16  bin_pt=14  quantization=Truncate  overflow=Wrap  dbl_ovrd=off  block_type=mux
  Mux3 : xbsIndex_r4/Mux  inputs=5  en=off  latency=1  precision=Full  arith_type=Unsigned  n_bits=16  bin_pt=14  quantization=Truncate  overflow=Wrap  dbl_ovrd=off  block_type=mux
  Mux4 : xbsIndex_r4/Mux  inputs=5  en=off  latency=1  precision=Full  arith_type=Unsigned  n_bits=16  bin_pt=14  quantization=Truncate  overflow=Wrap  dbl_ovrd=off  block_type=mux
  RSlice1 : xbsIndex_r4/Slice  nbits=3  boolean_output=off  mode=Upper Bit Location + Width  bit1=0  base1=MSB of Input  bit0=0  base0=LSB of Input  dbl_ovrd=off  block_type=slice
      settings: block_version=VER_STRING_GOES_HERE
  RSlice7 : xbsIndex_r4/Slice  nbits=7  boolean_output=off  mode=Lower Bit Location + Width  bit1=0  base1=MSB of Input  bit0=0  base0=LSB of Input  dbl_ovrd=off  block_type=slice
      settings: block_version=VER_STRING_GOES_HERE
  Relational{1..5,16..17} (7 alike) : xbsIndex_r4/Relational  mode=a=b  op_type=Bool  en=off  latency=0  dbl_ovrd=off  block_type=relational
  Scope1 : Scope  NumInputPorts=8
  Scope2 : Scope  NumInputPorts=8
  Scope3 : Scope  NumInputPorts=10
  Shift2 : xbsIndex_r4/Shift  shift_dir=Right  shift_bits=5  en=off  latency=0  precision=Full  arith_type="Signed  (2's comp)"  n_bits=16  bin_pt=14  quantization=Truncate  overflow=Wrap  dbl_ovrd=off  block_type=shift
  Single Port RAM5 : xbsIndex_r4/Single Port RAM  depth=96  initVector=exp_e4  distributed_mem=Block RAM  write_mode=Read After Write  rst=off  init_reg=0  en=off  latency=1  optimize=Area  dbl_ovrd=off  block_type=spram
  Single Port RAM6 : xbsIndex_r4/Single Port RAM  depth=96  initVector=exp_e3  distributed_mem=Block RAM  write_mode=Read After Write  rst=off  init_reg=0  en=off  latency=1  optimize=Area  dbl_ovrd=off  block_type=spram
  Single Port RAM7 : xbsIndex_r4/Single Port RAM  depth=96  initVector=exp_e2  distributed_mem=Block RAM  write_mode=Read After Write  rst=off  init_reg=0  en=off  latency=1  optimize=Area  dbl_ovrd=off  block_type=spram
  Single Port RAM8 : xbsIndex_r4/Single Port RAM  depth=96  initVector=exp_e1  distributed_mem=Block RAM  write_mode=Read After Write  rst=off  init_reg=0  en=off  latency=1  optimize=Area  dbl_ovrd=off  block_type=spram
  Single Port RAM9 : xbsIndex_r4/Single Port RAM  depth=96  initVector=exp_e0  distributed_mem=Block RAM  write_mode=Read After Write  rst=off  init_reg=0  en=off  latency=1  optimize=Area  dbl_ovrd=off  block_type=spram
  Slice1 : xbsIndex_r4/Slice  nbits=5  boolean_output=off  mode=Lower Bit Location + Width  bit1=0  base1=LSB of Input  bit0=0  base0=LSB of Input  dbl_ovrd=off  block_type=slice
  Slice3 : xbsIndex_r4/Slice  nbits=2  boolean_output=off  mode=Upper Bit Location + Width  bit1=0  base1=MSB of Input  bit0=0  base0=LSB of Input  dbl_ovrd=off  block_type=slice
  const : xbsIndex_r4/Constant  const=0  gui_display_data_type=Fixed-point  arith_type=Unsigned  n_bits=7  bin_pt=0  preci_type=Single  exp_width=8  frac_width=24  explicit_period=on  period=1  equ=P=C  opselect=C  inp2=PCIN>>17  opr=+  inp1=P  carry=CIN  dbl_ovrd=off  block_type=constant
      settings: block_version=VER_STRING_GOES_HERE
  x : xbsIndex_r4/Constant  const=8000000  gui_display_data_type=Fixed-point  arith_type=Unsigned  n_bits=24  bin_pt=0  preci_type=Single  exp_width=8  frac_width=24  explicit_period=on  period=1  equ=P=C  opselect=C  inp2=PCIN>>17  opr=+  inp1=P  carry=CIN  dbl_ovrd=off  block_type=constant
      settings: block_version=VER_STRING_GOES_HERE
  z1 : xbsIndex_r4/Delay  rst=off  infoeditControl=Selection of Reset will increase slice count due to use of real FFs and instead of SRLs  en=off  latency=3  reg_retiming=on  dbl_ovrd=off  block_type=delay
      settings: block_version=8.2-EVAL
  z{2,4..13,15,17..18,20..24} (19 alike) : xbsIndex_r4/Delay  rst=off  infoeditControl=Selection of Reset will increase slice count due to use of real FFs and instead of SRLs  en=off  latency=1  reg_retiming=on  dbl_ovrd=off  block_type=delay
      settings: block_version=8.2-EVAL
  z14 : xbsIndex_r4/Delay  rst=off  infoeditControl=Selection of Reset will increase slice count due to use of real FFs and instead of SRLs  en=off  latency=2  reg_retiming=on  dbl_ovrd=off  block_type=delay
      settings: block_version=8.2-EVAL
  z3 : xbsIndex_r4/Delay  rst=off  infoeditControl=Selection of Reset will increase slice count due to use of real FFs and instead of SRLs  en=off  latency=4  reg_retiming=on  dbl_ovrd=off  block_type=delay
      settings: block_version=8.2-EVAL
  Out : Outport
  wires:
  AddSub6/1 -> z17/1
  m_en/1 -> Relational17/1
  z12/1 -> Mux3/3, Scope3/3, Mux4/4
  z11/1 -> Mux4/5, Mux3/4, Scope3/4
  m_addr/1 -> RSlice7/1, RSlice1/1
  z10/1 -> Mux3/5, Scope3/5
  Constant2/1 -> Mux2/3
  Logical2/1 -> Single Port RAM7/3, Mux12/1
  z2/1 -> AddSub6/1, Scope1/6
  Single Port RAM8/1 -> z13/1
  Logical3/1 -> Mux13/1, Single Port RAM8/3
  Force_vol/1 -> Relational16/1, Slice1/1, Scope1/1, Slice3/1
  z20/1 -> z1/1, Scope1/2
  Single Port RAM9/1 -> z15/1
  Constant/1 -> Relational1/2
  Constant10/1 -> Mux3/6
  Logical/1 -> Scope2/2, Single Port RAM5/3, Mux10/1
  z1/1 -> Mult3/2, Scope1/4
  const/1 -> Relational16/2
  AddSub5/1 -> z23/1
  Mux4/1 -> z14/1, Scope3/7, AddSub5/2
  addr/1 -> z4/1
  Logical4/1 -> Single Port RAM9/3, Mux14/1
  RSlice1/1 -> Relational1/1, Relational5/1, Relational4/1, Relational3/1, Relational2/1
  Relational4/1 -> Logical3/2
  z9/1 -> Mux14/2
  Mux11/1 -> Single Port RAM6/1
  Constant3/1 -> Relational2/2
  Single Port RAM5/1 -> Scope2/3, z10/1
  z8/1 -> Mux13/2
  CMD_Firprg_1/1 -> Relational17/2
  z6/1 -> Mux11/2
  z5/1 -> Mux10/2
  Mux10/1 -> Scope2/1, Single Port RAM5/1
  m_data/1 -> Single Port RAM5/2, Single Port RAM6/2, Single Port RAM7/2, Single Port RAM9/2, Single Port RAM8/2
  Mux13/1 -> Single Port RAM8/1
  z14/1 -> z3/1
  Shift2/1 -> Mult3/1, Scope1/3
  Constant4/1 -> Relational3/2
  z7/1 -> Mux12/2
  Mux12/1 -> Single Port RAM7/1
  Mux3/1 -> Scope3/6, AddSub5/1
  Slice3/1 -> Convert5/1
  Constant5/1 -> Relational4/2
  Relational3/1 -> Logical2/2
  Logical1/1 -> Single Port RAM6/3, Mux11/1
  Relational17/1 -> Logical/1, Logical4/1, Logical3/1, Logical2/1, Logical1/1
  RSlice7/1 -> Mux11/3, Mux12/3, Mux14/3, Mux13/3, Mux10/3
  Constant6/1 -> Relational5/2
  Relational5/1 -> Logical4/2
  z15/1 -> Mux4/2
  Single Port RAM6/1 -> z11/1
  Single Port RAM7/1 -> z12/1
  Relational16/1 -> Mux2/1
  z13/1 -> Mux4/3, Mux3/2, Scope3/2
  Mult3/1 -> z2/1
  Convert5/1 -> Mux2/2
  Constant1/1 -> Mux4/6
  Relational2/1 -> Logical1/2
  Relational1/1 -> Logical/2
  z4/1 -> z7/1, z9/1, z8/1, z6/1, z5/1
  Mux14/1 -> Single Port RAM9/1
  z3/1 -> z24/1
  z18/1 -> Mux4/1, Mux3/1, Scope3/1
  Mux2/1 -> z18/1
  z21/1 -> z20/1
  Slice1/1 -> z22/1
  z22/1 -> z21/1
  z23/1 -> Shift2/1
  z24/1 -> AddSub6/2, Scope1/7
  z17/1 -> Out/1, Scope1/8

== system mapp_4_fir_4_str/mashinka_0/Force_str0/PARAMETERS/Subsystem1/Subsystem ==
  In1 : Inport
  Convert : xbsIndex_r4/Convert  gui_display_data_type=Boolean  arith_type=Boolean  n_bits=16  bin_pt=14  float_type=Single  exp_bits=8  fraction_bits=24  quantization=Truncate  overflow=Wrap  en=off  latency=0  pipeline=off  dbl_ovrd=off  block_type=convert
  Delay8 : xbsIndex_r4/Delay  rst=off  infoeditControl=Selection of Reset will increase slice count due to use of real FFs and instead of SRLs  en=off  latency=1  reg_retiming=off  dbl_ovrd=off  block_type=delay
  Delay9 : xbsIndex_r4/Delay  rst=off  infoeditControl=Selection of Reset will increase slice count due to use of real FFs and instead of SRLs  en=off  latency=1  reg_retiming=off  dbl_ovrd=off  block_type=delay
  Logical : xbsIndex_r4/Logical  logical_function=XOR  inputs=2  en=off  latency=0  precision=Full  arith_type=Unsigned  n_bits=16  bin_pt=0  align_bp=on  dbl_ovrd=off  block_type=logical
  Logical1 : xbsIndex_r4/Logical  logical_function=AND  inputs=2  en=off  latency=0  precision=Full  arith_type=Unsigned  n_bits=16  bin_pt=0  align_bp=on  dbl_ovrd=off  block_type=logical
  Logical2 : xbsIndex_r4/Logical  logical_function=AND  inputs=2  en=off  latency=0  precision=Full  arith_type=Unsigned  n_bits=16  bin_pt=0  align_bp=on  dbl_ovrd=off  block_type=logical
  Scope1 : Scope  NumInputPorts=8
  rise : Outport
  fall : Outport  Port=2
  wires:
  Delay8/1 -> Convert/1
  In1/1 -> Delay8/1
  Logical2/1 -> fall/1, Scope1/3
  Logical1/1 -> rise/1, Scope1/2
  Logical/1 -> Logical1/2, Logical2/1
  Delay9/1 -> Logical/2, Logical2/2
  Convert/1 -> Logical/1, Delay9/1, Scope1/1, Logical1/1
